simulink subsystem "edge1x1_simple_asSubsystem"  (R2021a)
settings: Solver=VariableStepAuto  StartTime=0.0  StopTime=10.0  RelTol=1e-3
libraries: simulink x1
settings Model: Creator=phill  LastModifiedBy=phill

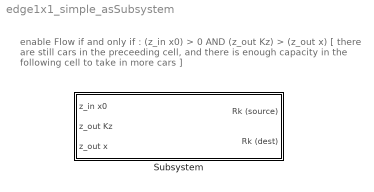
== system edge1x1_simple_asSubsystem ==
  note: enable Flow if and only if : (z_in x0) > 0 AND (z_out Kz) > (z_out x)
      | [ there are still cars in the preceeding cell, and there is enough capacity
      | in the following cell to take in more cars ]
  Subsystem : Subsystem  mask{Rk=1}
      mask prompts: Rk "Rk (fixed flowrate, used when the flow is enabled)"
      mask help: This block serves to establish a flow between two Street Lane Segments. To archieve this, it connects one source-cell [z_in] to one destination-cell [z_out], and prompts a flow of cars with the rate Rk (Parameter) if and only if there are still cars at the end of [z_out] avaiable and if the capacity of [z_out] is not yet surpassed, i.e. (z_in x0 > 0 AND z_out Kz > z_out x), otherwise the flow is reduced to 0.
      mask Display:
      | disp('Simple Edge 1x1 \n\n');
      | disp(['Rk = ', get_param(gcb,'Rk')])

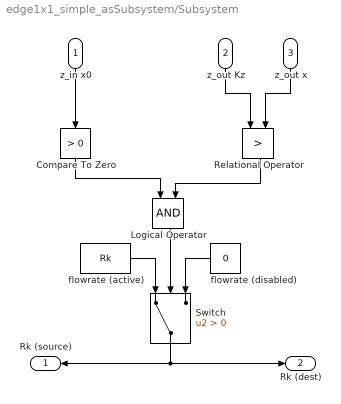
== system edge1x1_simple_asSubsystem/Subsystem ==
  z_in x0 : Inport
  z_out Kz : Inport  Port=2
  z_out x : Inport  Port=3
  Compare To Zero : simulink/Logic and Bit Operations/Compare To Zero  relop=>  OutDataTypeStr=boolean
  Logical Operator : Logic  AllPortsSameDT=off  OutDataTypeStr=boolean
  Relational Operator : RelationalOperator  Operator=>  OutDataTypeStr=boolean  RndMeth=Simplest
  Switch : Switch  Criteria=u2 > Threshold
  flowrate (active) : Constant  Value=Rk
  flowrate (disabled) : Constant  Value=0
  Rk (source) : Outport
  Rk (dest) : Outport  Port=2
  wires:
  flowrate (disabled)/1 -> Switch/3
  z_in x0/1 -> Compare To Zero/1
  Relational Operator/1 -> Logical Operator/2
  flowrate (active)/1 -> Switch/1
  Switch/1 -> Rk (dest)/1, Rk (source)/1
  z_out Kz/1 -> Relational Operator/1
  Logical Operator/1 -> Switch/2
  z_out x/1 -> Relational Operator/2
  Compare To Zero/1 -> Logical Operator/1
